simulink model "GANTRY_SYSID"  (R2024b)
settings: Solver=FixedStepAuto  StartTime=0.0  StopTime=inf  FixedStep=1/200  RelTol=1e-3  EnableMultiTasking=on
libraries: mbedblockslib x8
settings Model: ExtModeTrigDuration=10  Creator=patri  LastModifiedBy=Jaylen
settings SolverCC: AutoInsertRateTranBlk=on
settings OptimizationCC: EnhancedBackFolding=on  PassReuseOutputArgsAs=Individual arguments  ZeroExternalMemoryAtStartup=off  ZeroInternalMemoryAtStartup=off  MaxStackSize=64  OptimizeBlockOrder=speed  DifferentSizesBufferReuse=on  OptimizationCustomize=off  EfficientTunableParamExpr=on
settings DebuggingCC: ParameterTunabilityLossMsg=error
settings HardwareCC: ProdBitPerPointer=32  ProdBitPerSizeT=32  ProdBitPerPtrDiffT=32  ProdLargestAtomicInteger=Long  ProdLargestAtomicFloat=Double  ProdWordSize=32  ProdLongLongMode=on  ProdHWDeviceType=ARM Compatible->ARM Cortex-M
settings SFSimCC: MATLABDynamicMemAlloc=off
settings RTWCC: Description=Embedded Coder  SystemTargetFile=ert.tlc  HardwareBoard=STM32 Nucleo F767ZI  TemplateMakefile=ert_default_tmf  Toolchain=GNU Tools for ARM Embedded Processors
settings CodeAppCC: ForceParamTrailComments=on  IgnoreCustomStorageClasses=off  OperatorAnnotations=on  SimulinkDataObjDesc=on  SFDataObjDesc=on  InsertBlockDesc=on
settings ERTTargetCC: ExtModeTransport=3  ExtModeStaticAlloc=on  ExtModeStaticAllocSize=10000  ExtModeMexFile=ext_xcp  ExtModeIntrfLevel=Level2 - Open  InlinedParameterPlacement=Hierarchical

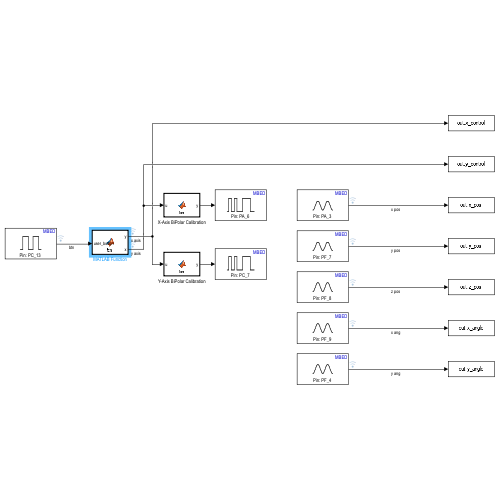
[thumbnail: Simulink's stored preview of the top-level diagram]
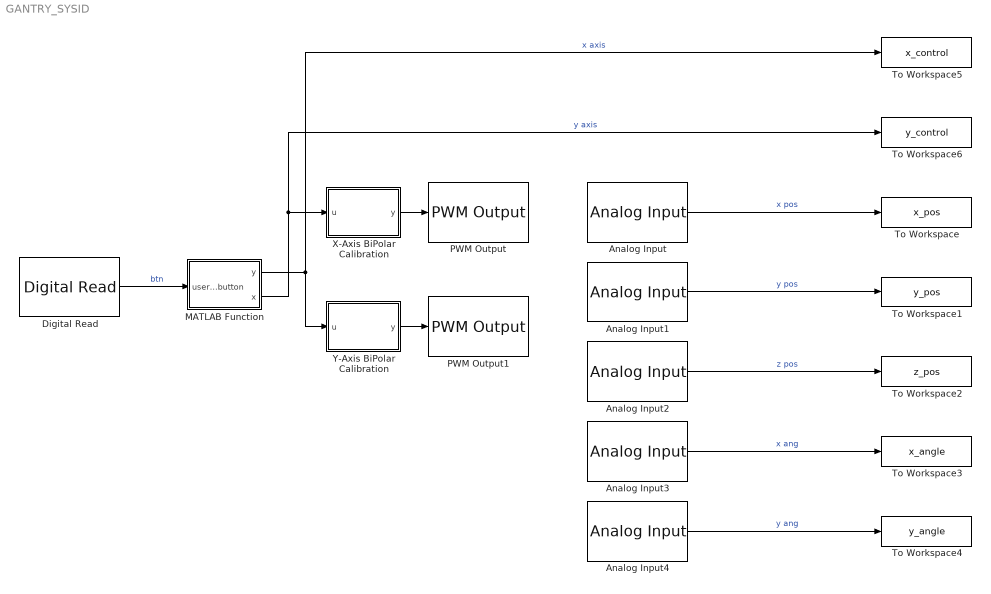
== system GANTRY_SYSID ==
  Analog Input : mbedblockslib/Analog Input  Pin=PA_3  ReadResultsOnly=off  ConversionTriggerSource=Software  ExternalTriggerType=uint32( 0 )  OutputDataType=double  EnableConversionCompleteNotify=off  EnableOuputStatus=off  SampleTime=-1
      settings: LibrarySourceBlock=stmnucleorootlib/Common/Analog Input
  Analog Input1 : mbedblockslib/Analog Input  Pin=PF_7  ReadResultsOnly=off  ConversionTriggerSource=Software  ExternalTriggerType=uint32( 0 )  OutputDataType=double  EnableConversionCompleteNotify=off  EnableOuputStatus=off  SampleTime=-1
      settings: LibrarySourceBlock=stmnucleorootlib/Common/Analog Input
  Analog Input2 : mbedblockslib/Analog Input  Pin=PF_8  ReadResultsOnly=off  ConversionTriggerSource=Software  ExternalTriggerType=uint32( 0 )  OutputDataType=double  EnableConversionCompleteNotify=off  EnableOuputStatus=off  SampleTime=-1
      settings: LibrarySourceBlock=stmnucleorootlib/Common/Analog Input
  Analog Input3 : mbedblockslib/Analog Input  Pin=PF_9  ReadResultsOnly=off  ConversionTriggerSource=Software  ExternalTriggerType=uint32( 0 )  OutputDataType=double  EnableConversionCompleteNotify=off  EnableOuputStatus=off  SampleTime=-1
      settings: LibrarySourceBlock=stmnucleorootlib/Common/Analog Input
  Analog Input4 : mbedblockslib/Analog Input  Pin=PF_4  ReadResultsOnly=off  ConversionTriggerSource=Software  ExternalTriggerType=uint32( 0 )  OutputDataType=double  EnableConversionCompleteNotify=off  EnableOuputStatus=off  SampleTime=-1
      settings: LibrarySourceBlock=stmnucleorootlib/Common/Analog Input
  Digital Read : mbedblockslib/Digital Read  Pin=PC_13  Direction=input  SampleTime=-1
      settings: LibrarySourceBlock=stmnucleorootlib/Common/Digital Read
  MATLAB Function : MATLAB Function  TreatAsAtomicUnit=on
  PWM Output : mbedblockslib/PWM Output  Pin=PA_6  EnableInputFrequency=off  InitialFrequency=10000  InitialDutyCycle=57.6  NotificationType=None
      settings: LibrarySourceBlock=stmnucleorootlib/Common/PWM Output
  PWM Output1 : mbedblockslib/PWM Output  Pin=PC_7  EnableInputFrequency=off  InitialFrequency=10000  InitialDutyCycle=57.6  NotificationType=None
      settings: LibrarySourceBlock=stmnucleorootlib/Common/PWM Output
  To Workspace : ToWorkspace  VariableName=x_pos  SaveFormat=Timeseries  SampleTime=-1
  To Workspace1 : ToWorkspace  VariableName=y_pos  SaveFormat=Timeseries  SampleTime=-1
  To Workspace2 : ToWorkspace  VariableName=z_pos  SaveFormat=Timeseries  SampleTime=-1
  To Workspace3 : ToWorkspace  VariableName=x_angle  SaveFormat=Timeseries  SampleTime=-1
  To Workspace4 : ToWorkspace  VariableName=y_angle  SaveFormat=Timeseries  SampleTime=-1
  To Workspace5 : ToWorkspace  VariableName=x_control  SaveFormat=Timeseries  SampleTime=-1
  To Workspace6 : ToWorkspace  VariableName=y_control  SaveFormat=Timeseries  SampleTime=-1
  X-Axis BiPolar Calibration : MATLAB Function  TreatAsAtomicUnit=on
  Y-Axis BiPolar Calibration : MATLAB Function  TreatAsAtomicUnit=on
  wires:
  Analog Input4/1 -> To Workspace4/1  "y ang"
  Analog Input2/1 -> To Workspace2/1  "z pos"
  Digital Read/1 -> MATLAB Function/1(user_button)  "btn"
  Analog Input/1 -> To Workspace/1  "x pos"
  Analog Input1/1 -> To Workspace1/1  "y pos"
  Analog Input3/1 -> To Workspace3/1  "x ang"
  X-Axis BiPolar Calibration/1(y) -> PWM Output/1
  Y-Axis BiPolar Calibration/1(y) -> PWM Output1/1
  MATLAB Function/2(x) -> To Workspace6/1, X-Axis BiPolar Calibration/1(u)  "y axis"
  MATLAB Function/1(y) -> To Workspace5/1, Y-Axis BiPolar Calibration/1(u)  "x axis"

== matlab function GANTRY_SYSID/MATLAB Function ==
  data: user_button input; y output; x output
function [y, x]= fcn(user_button)

persistent i m button_pressed

if isempty(m)
    m = 0;
    i = 0;
    button_pressed = 0;
end

Fs = 200;

if user_button == 1
    button_pressed = 1;
end

y = 0;
x = 0;
if button_pressed == 1
    if m == 0
        if i < 1*Fs
            x = 0;
        elseif i < 8*Fs
            x = 10;
        else
            x = 0;
            m = 1;
            i = 0;
            button_pressed = 0;
        end
    elseif m == 1
        if i < 1*Fs
            x = 0;
        elseif i < 8*Fs
            x = -10;
        else
            x = 0;
            m = 2;
            i = 0;
            button_pressed = 0;
        end
    elseif m == 2
        if i < 1*Fs
            y = 0;
        elseif i < 8*Fs
            y = 10;
        else
            y = 0;
            m = 3;
            i = 0;
            button_pressed = 0;
        end
    elseif m == 3
        if i < 1*Fs
            y = 0;
        elseif i < 8*Fs
            y = -10;
        else
            y = 0;
            m = 4;
            i = 0;
            button_pressed = 0;
        end
    else
        % Do Nothing
        x = 0;
        y = 0;
    end

    i = i + 1;
end

end

== matlab function GANTRY_SYSID/Y-Axis BiPolar Calibration ==
  data: u input; y output
function y = fcn(u)

y = 3.41*u + 59.49;

== matlab function GANTRY_SYSID/X-Axis BiPolar Calibration ==
  data: u input; y output
function y = fcn(u)

y = 2.758*u + 63.834;
